simulink model "battery_charger"  (R2024b)
settings: Solver=VariableStepAuto  StartTime=0.0  StopTime=2  RelTol=1e-3
undefined symbols (not defined in the file): Ion, Lithium
libraries: spsSeriesRLCBranchLib x3, spsDiodeLib x3, spsBatteryLib x1, spsIGBTLib x1, spsLinearTransformerLib x1, eePwmGenerator x1, spsPVArrayLib x1, spspowerguiLib x1
settings Model: SimulationMode=accelerator  Creator=himan  LastModifiedBy=himan
settings ModelReferenceCC: EnableRefExpFcnMdlSchedulingChecks=on
settings RTWCC: GPUComputeCapability=3.5

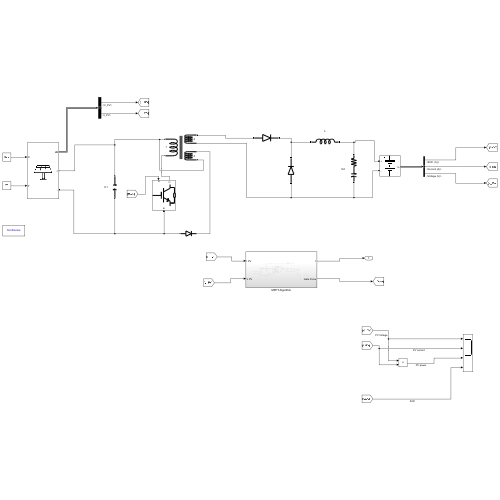
[thumbnail: Simulink's stored preview of the top-level diagram]
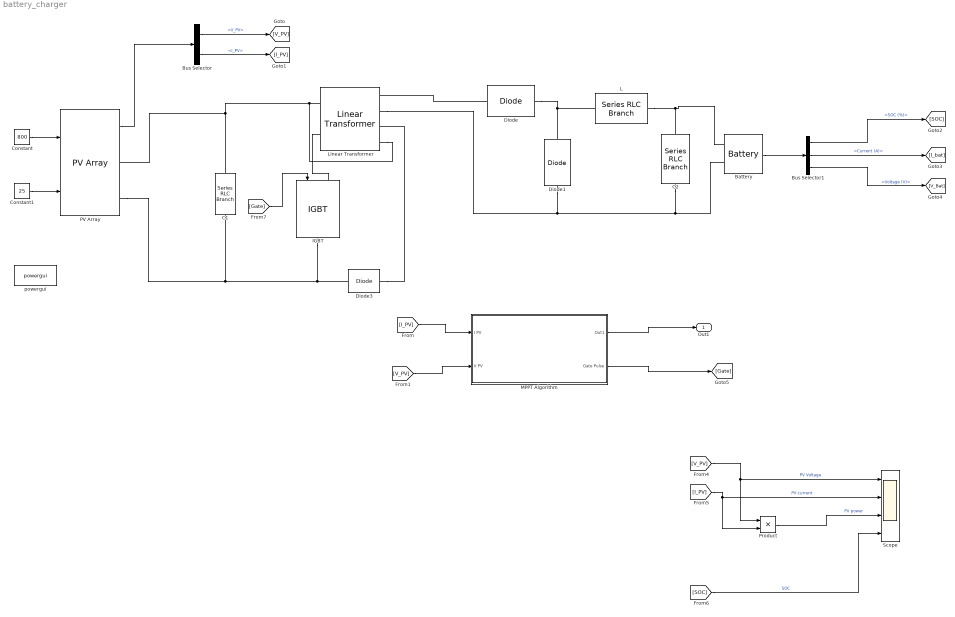
== system battery_charger ==
  Battery : spsBatteryLib/Battery  BatType=Lithium-Ion  NomV=320  NomQ=126  SOC=40  Batt_Tr=30  PresetModel=on  MaxQ=126  MinV=240  FullV=372.4759  Dis_rate=54.7826  R=0.025397  Normal_OP=113.9478  expZone="[345.7235      6.190435]"
  Bus Selector : BusSelector  OutputSignals=V_PV,I_PV
  Bus Selector1 : BusSelector  OutputSignals=SOC (%),Current (A),Voltage (V)
  C1 : spsSeriesRLCBranchLib/Series RLC Branch  LConnTagsString=__new0  RConnTagsString=__new0  BranchType=C  Resistance=0  Inductance=0  SetiL0=off  InitialCurrent=0  Capacitance=1e-3  Setx0=off  InitialVoltage=0  Measurements=None
  C2 : spsSeriesRLCBranchLib/Series RLC Branch  LConnTagsString=__new0  RConnTagsString=__new0  BranchType=RC  Resistance=0.001  Inductance=0  SetiL0=off  InitialCurrent=0  Capacitance=1e-3  Setx0=off  InitialVoltage=0  Measurements=None
  Constant : Constant  Value=800
  Constant1 : Constant  Value=25
  Diode : spsDiodeLib/Diode  Ron=0.001  Lon=0  Vf=0.8  IC=0  UseSnubber=0  Rs=inf  Cs=0  Measurements=off
  Diode1 : spsDiodeLib/Diode  Ron=0.001  Lon=0  Vf=0.8  IC=0  UseSnubber=0  Rs=inf  Cs=0  Measurements=off
  Diode3 : spsDiodeLib/Diode  Ron=0.001  Lon=0  Vf=0.8  IC=0  UseSnubber=0  Rs=inf  Cs=0  Measurements=off
  IGBT : spsIGBTLib/IGBT  Ron=1e-3  Lon=0  Vf=1  Tf=1e-6  Tt=2e-6  IC=0  Rs=1e5  Cs=inf  Measurements=off
  L : spsSeriesRLCBranchLib/Series RLC Branch  LConnTagsString=__new0  RConnTagsString=__new0  BranchType=L  Resistance=0  Inductance=1e-1  SetiL0=off  InitialCurrent=0  Capacitance=1e-6  Setx0=off  InitialVoltage=0  Measurements=None
  Linear Transformer : spsLinearTransformerLib/Linear Transformer  UNITS=SI  NominalPower=[ 250 20e3 ]  winding1=[40 0 0]  winding2=[440 0 0]  ThreeWindings=on  winding3=[40 0 0]  RmLm=[inf 10e-3]  Measurements=Magnetization current  DataType=on
  MPPT Algorithm : Subsystem
  PV Array : spsPVArrayLib/PV Array  Npar=1  Nser=1  PlotType=array @ 25 deg.C & specified irradiances  S_vec="[ 1000  800 ]"  Temp_C_vec="[ 45 25  ]"  ModuleName=User-defined  PlotWhenSelected=off  Pm=535.392  Ncell=144  Voc=49.4  Isc=13.56  Vm=41.6  Im=12.87  beta_Voc_pc=-0.27  alpha_Isc_pc=0.05  beta_Voc=-0.13338  alpha_Isc=0.00678  IL=13.5812  I0=1.2378e-11  nI=0.48183  Rsh=307.5281  Rs=0.17005  RobustModel=off  RobustCellTemperature=313.3991  BAL=on  Tc=1e-6  Tfilter=5e-5
  Product : Product
  Scope : Scope  NumInputPorts=4
  powergui : spspowerguiLib/powergui  Priority=1  SimulationMode=Continuous  SampleTime=1e-5  frequency=60  Iterations=50  frequencyindice=0  Pbase=100e6  ErrMax=1e-4  UnitsV=kV  UnitsW=MW  buscounter=0  FunctionMessages=off  echomessages=off  EnableUseOfTLC=off  CurrentSourceSwitches=off  DisableSnubberDevices=off  DisableRonSwitches=off  DisableVfSwitches=off  DisplayEquations=off  AutomaticDiscreteSolvers=off  SolverType=Tustin/Backward Euler (TBE)  Interpol=off  ExternalGateDelay=off  methode=off  Ts=100  x0status=blocks  SPID=on  SwTol=0  HookPort=off  NonlinearTolerance=1e-4  nMaxIteration=100  ContinueOnMaxIteration=off  RestoreLinks=warning  ResistiveCurrentMeasurement=off  Frange=[0:2:500]  Ylog=off  Xlog=on  ShowGrid=off  save=off  variable=ZData  structure=0  ZoomFFT=off  StartTime=0.0  cycles=1  DisplayStyle=1  fundamental=60  FreqAxis=off  MaxFrequency=1000  frequencyindicesteady=1  RmsSteady=1  display=off
  Out1 : Outport
  wires:
  Constant/1 -> PV Array/1
  Constant1/1 -> PV Array/2
  PV Array/1 -> Bus Selector/1
  Bus Selector/1 -> [V_PV]  "<V_PV>"
  Bus Selector/2 -> [I_PV]  "<I_PV>"
  [V_PV] -> Product/1, Scope/1  "PV Voltage"
  [I_PV] -> Product/2, Scope/2  "PV current"
  Bus Selector1/1 -> [SOC]  "<SOC (%)>"
  Bus Selector1/2 -> [I_bat]  "<Current (A)>"
  Bus Selector1/3 -> [V_Bat]  "<Voltage (V)>"
  [SOC] -> Scope/4  "SOC"
  [Gate] -> IGBT/1
  Battery/1 -> Bus Selector1/1
  MPPT Algorithm/1(Out1) -> Out1/1
  MPPT Algorithm/2(Gate Pulse) -> [Gate]
  Product/1 -> Scope/3  "PV power"
  [V_PV] -> MPPT Algorithm/2(V PV)
  [I_PV] -> MPPT Algorithm/1(I PV)
  connections:
  C1/LConn1 -- Linear Transformer/LConn1 -- Linear Transformer/RConn4 -- PV Array/RConn1
  PV Array/RConn2 -- Diode3/LConn1 -- IGBT/RConn1 -- C1/RConn1
  C2/LConn1 -- Battery/LConn1 -- L/LConn1
  C2/RConn1 -- Battery/LConn2 -- Linear Transformer/RConn2 -- Diode1/LConn1
  Linear Transformer/LConn2 -- IGBT/LConn1
  Diode/LConn1 -- Linear Transformer/RConn1
  Diode/RConn1 -- Diode1/RConn1 -- L/RConn1
  Diode3/RConn1 -- Linear Transformer/RConn3

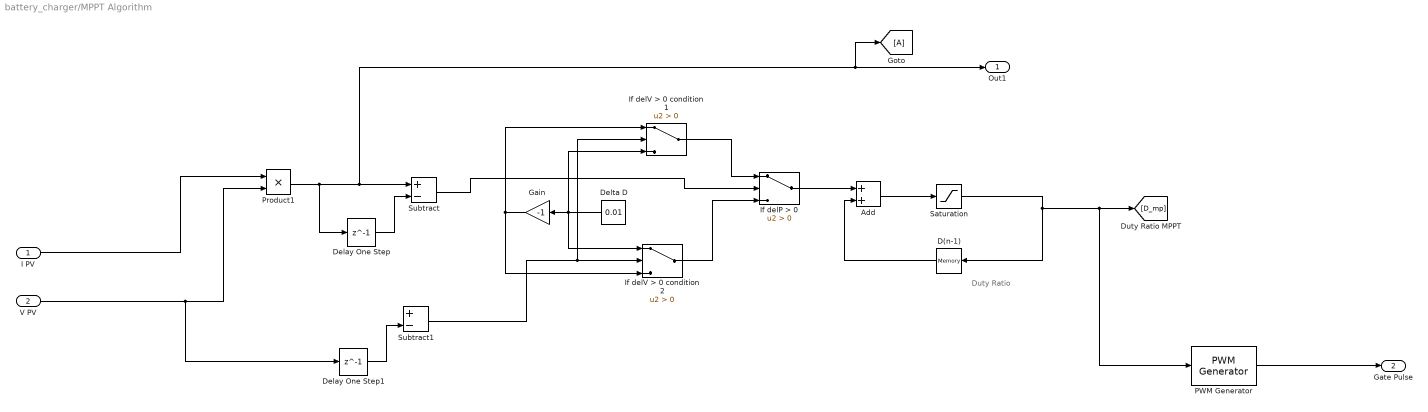
== system battery_charger/MPPT Algorithm ==
  note: Duty Ratio
  I PV : Inport
  V PV : Inport  Port=2
  Add : Sum
  D(n-1) : Memory  InheritSampleTime=on
  Delay One Step : Delay  DelayLength=1
  Delay One Step1 : Delay  DelayLength=1
  Delta D : Constant  Value=0.01
  Gain : Gain  Gain=-1
  Goto : Goto
  "If delP > 0 " : Switch  Criteria=u2 > Threshold  SaturateOnIntegerOverflow=off  InputSameDT=off
  If delV > 0 condition 1 : Switch  Criteria=u2 > Threshold  SaturateOnIntegerOverflow=off  InputSameDT=off
  "If delV > 0 condition 2 " : Switch  Criteria=u2 > Threshold  SaturateOnIntegerOverflow=off  InputSameDT=off
  PWM Generator : eePwmGenerator/PWM Generator  CarrCount=Up  Tper=0.001  Tdelay=0  Ts=5e-5
  Product1 : Product
  Saturation : Saturate  UpperLimit=1  LowerLimit=0
  Subtract : Sum  Inputs=+-
  Subtract1 : Sum  Inputs=+-
  Out1 : Outport
  Gate Pulse : Outport  Port=2
  wires:
  Add/1 -> Saturation/1
  Delta D/1 -> "If delV > 0 condition 2 "/1, If delV > 0 condition 1/3, Gain/1
  Gain/1 -> "If delV > 0 condition 2 "/3, If delV > 0 condition 1/1
  Saturation/1 -> PWM Generator/1, [D_mp], D(n-1)/1
  Subtract/1 -> "If delP > 0 "/2
  Subtract1/1 -> If delV > 0 condition 1/2, "If delV > 0 condition 2 "/2
  "If delP > 0 "/1 -> Add/1
  "If delV > 0 condition 2 "/1 -> "If delP > 0 "/3
  Product1/1 -> Goto/1, Out1/1, Subtract/1, Delay One Step/1
  Delay One Step1/1 -> Subtract1/2
  D(n-1)/1 -> Add/2
  If delV > 0 condition 1/1 -> "If delP > 0 "/1
  Delay One Step/1 -> Subtract/2
  PWM Generator/1 -> Gate Pulse/1
  I PV/1 -> Product1/1
  V PV/1 -> Delay One Step1/1, Product1/2
